simulink model "robots"  (R2018a)
settings: Solver=VariableStepAuto  StartTime=0.0  StopTime=10.0  RelTol=1e-3
undefined symbols (not defined in the file): sigbuilder_block
settings Model: EnablePacing=on  Creator=U500304  LastModifiedBy=U500304

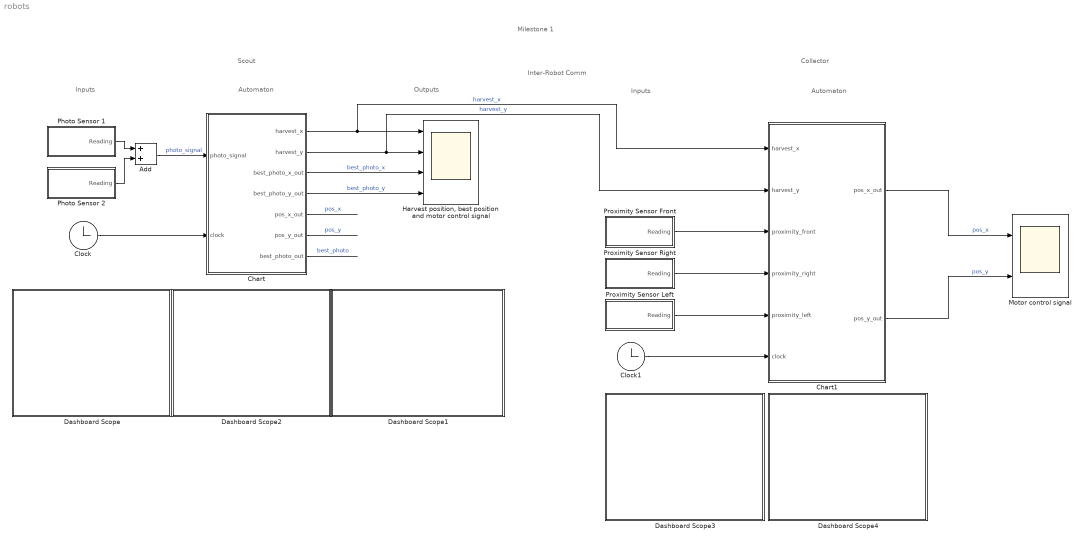
== system robots ==
  note: Inter-Robot
      | Comm
  note: Scout
  note: Milestone 1
  note: Inputs
  note: Automaton
  note: Outputs
  note: Inputs
  note: Collector
  note: Automaton
  Add : Sum
  Chart : Stateflow chart  TreatAsAtomicUnit=on
  Chart1 : Stateflow chart  TreatAsAtomicUnit=on
  Clock : Clock
  Clock1 : Clock
  Dashboard Scope : Subsystem  DialogController=hmiCreateDDGDialog  IsWebBlock=on  mask(MWDashboardBlock){webBlockId=c2b4710b-9c10-441f-91da-978dfb24ecfa, webBlockType=sdiscope, ShowInitialText=on, HMISrcModelName=scout}
      mask prompts: webBlockId "WebBlock Id"; webBlockType "WebBlock Type"; HMISrcModelName "Source Model"
      mask help: SimulinkHMI:dialogs:HMIScopeDialogDesc
      mask Help: helpview([docroot '/mapfiles/simulink.map'], 'hmi_scope')
      mask Display:
      | if strcmp(get_param(bdroot(gcb),'BlockDiagramType'), 'library')
      |     image([(matlabroot) '/toolbox/simulink/hmi/icons/DashboardScope.png']);
      | end
  Dashboard Scope1 : Subsystem  DialogController=hmiCreateDDGDialog  IsWebBlock=on  mask(MWDashboardBlock){webBlockId=2d41d672-6b82-41b2-afbb-9518b0dd4a4f, webBlockType=sdiscope, ShowInitialText=on, HMISrcModelName=scout}
      mask prompts: webBlockId "WebBlock Id"; webBlockType "WebBlock Type"; HMISrcModelName "Source Model"
      mask help: SimulinkHMI:dialogs:HMIScopeDialogDesc
      mask Help: helpview([docroot '/mapfiles/simulink.map'], 'hmi_scope')
      mask Display:
      | if strcmp(get_param(bdroot(gcb),'BlockDiagramType'), 'library')
      |     image([(matlabroot) '/toolbox/simulink/hmi/icons/DashboardScope.png']);
      | end
  Dashboard Scope2 : Subsystem  DialogController=hmiCreateDDGDialog  IsWebBlock=on  mask(MWDashboardBlock){webBlockId=ed7f14d0-e4f2-40fb-83fb-68689640cdf1, webBlockType=sdiscope, ShowInitialText=on, HMISrcModelName=scout}
      mask prompts: webBlockId "WebBlock Id"; webBlockType "WebBlock Type"; HMISrcModelName "Source Model"
      mask help: SimulinkHMI:dialogs:HMIScopeDialogDesc
      mask Help: helpview([docroot '/mapfiles/simulink.map'], 'hmi_scope')
      mask Display:
      | if strcmp(get_param(bdroot(gcb),'BlockDiagramType'), 'library')
      |     image([(matlabroot) '/toolbox/simulink/hmi/icons/DashboardScope.png']);
      | end
  Dashboard Scope3 : Subsystem  DialogController=hmiCreateDDGDialog  IsWebBlock=on  mask(MWDashboardBlock){webBlockId=b30215f1-102d-4ac5-97b6-32221d9819d8, webBlockType=sdiscope, ShowInitialText=on, HMISrcModelName=scout}
      mask prompts: webBlockId "WebBlock Id"; webBlockType "WebBlock Type"; HMISrcModelName "Source Model"
      mask help: SimulinkHMI:dialogs:HMIScopeDialogDesc
      mask Help: helpview([docroot '/mapfiles/simulink.map'], 'hmi_scope')
      mask Display:
      | if strcmp(get_param(bdroot(gcb),'BlockDiagramType'), 'library')
      |     image([(matlabroot) '/toolbox/simulink/hmi/icons/DashboardScope.png']);
      | end
  Dashboard Scope4 : Subsystem  DialogController=hmiCreateDDGDialog  IsWebBlock=on  mask(MWDashboardBlock){webBlockId=4fc18f5f-2100-4ee3-a4cf-c6ec907fe0c9, webBlockType=sdiscope, ShowInitialText=on, HMISrcModelName=scout}
      mask prompts: webBlockId "WebBlock Id"; webBlockType "WebBlock Type"; HMISrcModelName "Source Model"
      mask help: SimulinkHMI:dialogs:HMIScopeDialogDesc
      mask Help: helpview([docroot '/mapfiles/simulink.map'], 'hmi_scope')
      mask Display:
      | if strcmp(get_param(bdroot(gcb),'BlockDiagramType'), 'library')
      |     image([(matlabroot) '/toolbox/simulink/hmi/icons/DashboardScope.png']);
      | end
  "Harvest position, best position and motor control signal" : Scope  NumInputPorts=4
  Motor control signal : Scope  NumInputPorts=2
  Photo Sensor 1 : Subsystem  Tag=STV Subsys  LoadFcn=sigbuilder_block('load');  StartFcn=sigbuilder_block('start');  StopFcn=sigbuilder_block('stop');  ClipboardFcn=sigbuilder_block('clipboard');  mask(Sigbuilder block){tuvar=[0:10]}
      mask help: Simulink:masks:SigbuilderBlock_MD
      mask init:
      | if ~strcmp(get_param(bdroot(gcbh),'SimulationStatus'),'stopped') tuvar = sigbuilder_block('maskInit'); end
      settings: CopyFcn=sigbuilder_block('copy');  DeleteFcn=sigbuilder_block('delete');  ModelCloseFcn=sigbuilder_block('modelClose');  PreSaveFcn=sigbuilder_block('preSave');  PauseFcn=sigbuilder_block('pause');  ContinueFcn=sigbuilder_block('continue');  NameChangeFcn=sigbuilder_block('namechange');  OpenFcn=sigbuilder_block('open',[5.4 30 1141.2 522.6 ]);  CloseFcn=sigbuilder_block('close');
      mask Display: plot(0, 0, 100, 100,[2, 2, 32, 32, 2], [68, 8, 8, 68, 68],[32, 2], [38, 38], [32, 19, 2],[53, 60, 44], [32, 17, 17, 2],[16, 16, 31, 31]);txt = getActiveGroup(gcbh);text(2, 100, txt,'verticalAlignment', 'top');
  Photo Sensor 2 : Subsystem  Tag=STV Subsys  LoadFcn=sigbuilder_block('load');  StartFcn=sigbuilder_block('start');  StopFcn=sigbuilder_block('stop');  ClipboardFcn=sigbuilder_block('clipboard');  mask(Sigbuilder block){tuvar=[0:10]}
      mask help: Simulink:masks:SigbuilderBlock_MD
      mask init:
      | if ~strcmp(get_param(bdroot(gcbh),'SimulationStatus'),'stopped') tuvar = sigbuilder_block('maskInit'); end
      settings: CopyFcn=sigbuilder_block('copy');  DeleteFcn=sigbuilder_block('delete');  ModelCloseFcn=sigbuilder_block('modelClose');  PreSaveFcn=sigbuilder_block('preSave');  PauseFcn=sigbuilder_block('pause');  ContinueFcn=sigbuilder_block('continue');  NameChangeFcn=sigbuilder_block('namechange');  OpenFcn=sigbuilder_block('open',[5.4 30 1141.2 522.6 ]);  CloseFcn=sigbuilder_block('close');
      mask Display: plot(0, 0, 100, 100,[2, 2, 32, 32, 2], [68, 8, 8, 68, 68],[32, 2], [38, 38], [32, 19, 2],[53, 60, 44], [32, 17, 17, 2],[16, 16, 31, 31]);txt = getActiveGroup(gcbh);text(2, 100, txt,'verticalAlignment', 'top');
  Proximity Sensor Front : Subsystem  Tag=STV Subsys  LoadFcn=sigbuilder_block('load');  StartFcn=sigbuilder_block('start');  StopFcn=sigbuilder_block('stop');  ClipboardFcn=sigbuilder_block('clipboard');  mask(Sigbuilder block){tuvar=[0:10]}
      mask help: Simulink:masks:SigbuilderBlock_MD
      mask init:
      | if ~strcmp(get_param(bdroot(gcbh),'SimulationStatus'),'stopped') tuvar = sigbuilder_block('maskInit'); end
      settings: CopyFcn=sigbuilder_block('copy');  DeleteFcn=sigbuilder_block('delete');  ModelCloseFcn=sigbuilder_block('modelClose');  PreSaveFcn=sigbuilder_block('preSave');  PauseFcn=sigbuilder_block('pause');  ContinueFcn=sigbuilder_block('continue');  NameChangeFcn=sigbuilder_block('namechange');  OpenFcn=sigbuilder_block('open',[5.4 30 1141.2 522.6 ]);  CloseFcn=sigbuilder_block('close');
      mask Display: plot(0, 0, 100, 100,[2, 2, 32, 32, 2], [68, 8, 8, 68, 68],[32, 2], [38, 38], [32, 19, 2],[53, 60, 44], [32, 17, 17, 2],[16, 16, 31, 31]);txt = getActiveGroup(gcbh);text(2, 100, txt,'verticalAlignment', 'top');
  Proximity Sensor Left : Subsystem  Tag=STV Subsys  LoadFcn=sigbuilder_block('load');  StartFcn=sigbuilder_block('start');  StopFcn=sigbuilder_block('stop');  ClipboardFcn=sigbuilder_block('clipboard');  mask(Sigbuilder block){tuvar=[0:10]}
      mask help: Simulink:masks:SigbuilderBlock_MD
      mask init:
      | if ~strcmp(get_param(bdroot(gcbh),'SimulationStatus'),'stopped') tuvar = sigbuilder_block('maskInit'); end
      settings: CopyFcn=sigbuilder_block('copy');  DeleteFcn=sigbuilder_block('delete');  ModelCloseFcn=sigbuilder_block('modelClose');  PreSaveFcn=sigbuilder_block('preSave');  PauseFcn=sigbuilder_block('pause');  ContinueFcn=sigbuilder_block('continue');  NameChangeFcn=sigbuilder_block('namechange');  OpenFcn=sigbuilder_block('open',[5.4 30 1141.2 522.6 ]);  CloseFcn=sigbuilder_block('close');
      mask Display: plot(0, 0, 100, 100,[2, 2, 32, 32, 2], [68, 8, 8, 68, 68],[32, 2], [38, 38], [32, 19, 2],[53, 60, 44], [32, 17, 17, 2],[16, 16, 31, 31]);txt = getActiveGroup(gcbh);text(2, 100, txt,'verticalAlignment', 'top');
  Proximity Sensor Right : Subsystem  Tag=STV Subsys  LoadFcn=sigbuilder_block('load');  StartFcn=sigbuilder_block('start');  StopFcn=sigbuilder_block('stop');  ClipboardFcn=sigbuilder_block('clipboard');  mask(Sigbuilder block){tuvar=[0:10]}
      mask help: Simulink:masks:SigbuilderBlock_MD
      mask init:
      | if ~strcmp(get_param(bdroot(gcbh),'SimulationStatus'),'stopped') tuvar = sigbuilder_block('maskInit'); end
      settings: CopyFcn=sigbuilder_block('copy');  DeleteFcn=sigbuilder_block('delete');  ModelCloseFcn=sigbuilder_block('modelClose');  PreSaveFcn=sigbuilder_block('preSave');  PauseFcn=sigbuilder_block('pause');  ContinueFcn=sigbuilder_block('continue');  NameChangeFcn=sigbuilder_block('namechange');  OpenFcn=sigbuilder_block('open',[5.4 30 1141.2 522.6 ]);  CloseFcn=sigbuilder_block('close');
      mask Display: plot(0, 0, 100, 100,[2, 2, 32, 32, 2], [68, 8, 8, 68, 68],[32, 2], [38, 38], [32, 19, 2],[53, 60, 44], [32, 17, 17, 2],[16, 16, 31, 31]);txt = getActiveGroup(gcbh);text(2, 100, txt,'verticalAlignment', 'top');
  wires:
  Chart/6(pos_y_out) -> ?  "pos_y"
  Chart/5(pos_x_out) -> ?  "pos_x"
  Chart/2(harvest_y) -> Chart1/2(harvest_y), "Harvest position, best position and motor control signal"/2  "harvest_y"
  Chart/3(best_photo_x_out) -> "Harvest position, best position and motor control signal"/3  "best_photo_x"
  Chart/1(harvest_x) -> Chart1/1(harvest_x), "Harvest position, best position and motor control signal"/1  "harvest_x"
  Photo Sensor 2/1(Reading) -> Add/2
  Photo Sensor 1/1(Reading) -> Add/1
  Chart/4(best_photo_y_out) -> "Harvest position, best position and motor control signal"/4  "best_photo_y"
  Chart/7(best_photo_out) -> ?  "best_photo"
  Add/1 -> Chart/1(photo_signal)  "photo_signal"
  Clock/1 -> Chart/2(clock)
  Proximity Sensor Front/1(Reading) -> Chart1/3(proximity_front)
  Proximity Sensor Right/1(Reading) -> Chart1/4(proximity_right)
  Proximity Sensor Left/1(Reading) -> Chart1/5(proximity_left)
  Clock1/1 -> Chart1/6(clock)
  Chart1/1(pos_x_out) -> Motor control signal/1  "pos_x"
  Chart1/2(pos_y_out) -> Motor control signal/2  "pos_y"

== system robots/Dashboard Scope ==

== system robots/Dashboard Scope1 ==

== system robots/Dashboard Scope2 ==

== system robots/Dashboard Scope3 ==

== system robots/Dashboard Scope4 ==

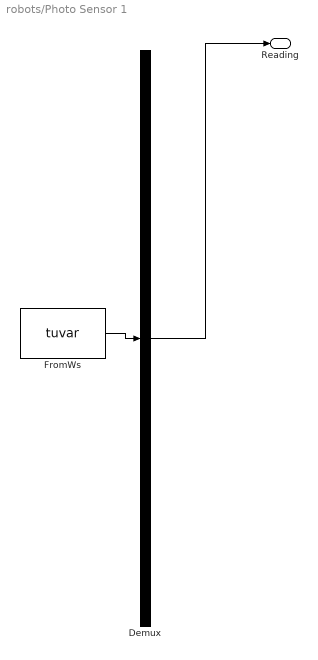
== system robots/Photo Sensor 1 ==
  Demux : Demux  Tag=STV Demux  Outputs=1
  FromWs : FromWorkspace  Tag=STV FromWs  VariableName=tuvar  SampleTime=0
      SigBuilderData=|
      | common.afterFinalStr = 'Extrapolate'
      | common.sampleTime = 0
      | dataSet.timeRange = [0 10]
      | dataSet.name = 'Photo Sensor'
      | sbobj.Groups.Name = 'Photo Sensor'
      | sbobj.Groups.Signals.Name = 'Reading'
      | sbobj.Groups.Signals.XData = [0 6 6 8 8 10]
      | sbobj.Groups.Signals.YData = [0 0 300 300 0 0]
  Reading : Outport  Tag=STV Outport
  wires:
  Demux/1 -> Reading/1
  FromWs/1 -> Demux/1

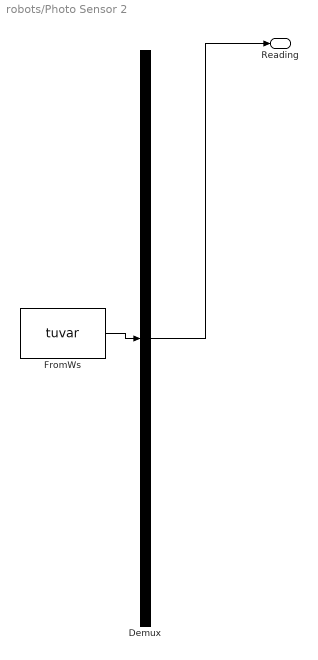
== system robots/Photo Sensor 2 ==
  Demux : Demux  Tag=STV Demux  Outputs=1
  FromWs : FromWorkspace  Tag=STV FromWs  VariableName=tuvar  SampleTime=0
      SigBuilderData=|
      | common.afterFinalStr = 'Extrapolate'
      | common.sampleTime = 0
      | dataSet.timeRange = [0 10]
      | dataSet.name = 'Photo Sensor'
      | sbobj.Groups.Name = 'Photo Sensor'
      | sbobj.Groups.Signals.Name = 'Reading'
      | sbobj.Groups.Signals.XData = [0 2 2 5 5 10]
      | sbobj.Groups.Signals.YData = [0 0 180 180 0 0]
  Reading : Outport  Tag=STV Outport
  wires:
  FromWs/1 -> Demux/1
  Demux/1 -> Reading/1

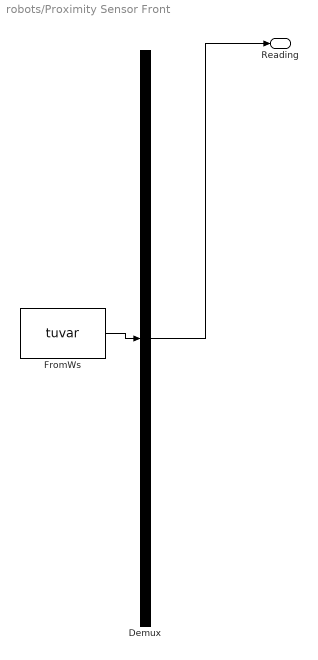
== system robots/Proximity Sensor Front ==
  Demux : Demux  Tag=STV Demux  Outputs=1
  FromWs : FromWorkspace  Tag=STV FromWs  VariableName=tuvar  SampleTime=0
      SigBuilderData=|
      | common.afterFinalStr = 'Extrapolate'
      | common.sampleTime = 0
      | dataSet.timeRange = [0 10]
      | dataSet.name = 'Proximity Front'
      | sbobj.Groups.Name = 'Proximity Front'
      | sbobj.Groups.Signals.Name = 'Reading'
      | sbobj.Groups.Signals.XData = [0 1 8 10]
      | sbobj.Groups.Signals.YData = [10 10 0 0]
  Reading : Outport  Tag=STV Outport
  wires:
  FromWs/1 -> Demux/1
  Demux/1 -> Reading/1

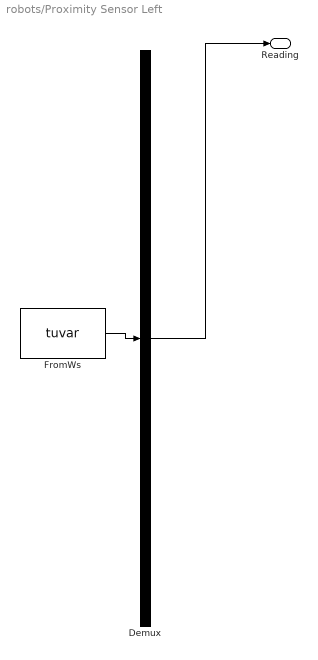
== system robots/Proximity Sensor Left ==
  Demux : Demux  Tag=STV Demux  Outputs=1
  FromWs : FromWorkspace  Tag=STV FromWs  VariableName=tuvar  SampleTime=0
      SigBuilderData=|
      | common.afterFinalStr = 'Extrapolate'
      | common.sampleTime = 0
      | dataSet.timeRange = [0 10]
      | dataSet.name = 'Proximity Left'
      | sbobj.Groups.Name = 'Proximity Left'
      | sbobj.Groups.Signals.Name = 'Reading'
      | sbobj.Groups.Signals.XData = [0 1 2 10]
      | sbobj.Groups.Signals.YData = [2 2 3 8.2]
  Reading : Outport  Tag=STV Outport
  wires:
  FromWs/1 -> Demux/1
  Demux/1 -> Reading/1

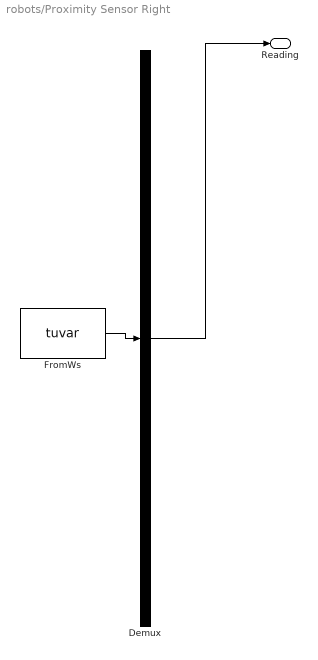
== system robots/Proximity Sensor Right ==
  Demux : Demux  Tag=STV Demux  Outputs=1
  FromWs : FromWorkspace  Tag=STV FromWs  VariableName=tuvar  SampleTime=0
      SigBuilderData=|
      | common.afterFinalStr = 'Extrapolate'
      | common.sampleTime = 0
      | dataSet.timeRange = [0 10]
      | dataSet.name = 'Proximity Right'
      | sbobj.Groups.Name = 'Proximity Right'
      | sbobj.Groups.Signals.Name = 'Reading'
      | sbobj.Groups.Signals.XData = [0 1 10]
      | sbobj.Groups.Signals.YData = [5 4.4 0.55]
  Reading : Outport  Tag=STV Outport
  wires:
  Demux/1 -> Reading/1
  FromWs/1 -> Demux/1

== stateflow chart robots/Chart1 ==
  settings: updateMethod=CONTINUOUS
  state Annoy
    state DriveForward
      du:
      pos_x_dot = 1;
      pos_y_dot = 0;
      pos_x_out = pos_x;
      pos_y_out = pos_y;
    state TurnLeft
      du:
      pos_x_dot = 1;
      pos_y_dot = 0;
      pos_x_out = pos_x;
      pos_y_out = pos_y;
    state TurnRight
      du:
      pos_x_dot = 1;
      pos_y_dot = 0;
      pos_x_out = pos_x;
      pos_y_out = pos_y;
    note: Tries to annoy other robots by pushing them using proximity sensor readings
    (default) -> Annoy.DriveForward
    TurnLeft -> Annoy.DriveForward [order 2] : [proximity_front < proximity_left]
    TurnRight -> Annoy.DriveForward [order 2] : [proximity_front < proximity_right]
    Annoy.DriveForward -> TurnRight [order 2] : [proximity_right < proximity_front]
    Annoy.DriveForward -> TurnLeft [order 1] : [proximity_left < proximity_front]
    TurnLeft -> TurnRight [order 1] : [proximity_right < proximity_left]
    TurnRight -> TurnLeft [order 1] : [proximity_left < proximity_right]
  state Harvest
    state DriveForward
      du:
      pos_x_dot = 0;
      pos_y_dot = 1;
      pos_x_out = pos_x;
      pos_y_out = pos_y;
    note: Drives to the given location of light
    (default) -> Harvest.DriveForward
  (default) -> Annoy : {
      | pos_x = 0;
      | pos_y = 0'
      | }
  Annoy -> Harvest : [harvest_x > -1 && harvest_y > -1]
  data: harvest_x input; harvest_y input; proximity_front input; proximity_right input; proximity_left input; clock input; pos_x local; pos_y local; pos_x_out output; pos_y_out output; target_dir_x local; target_dir_y local
  data pos_x settings: updateMethod=SF_CONTINUOUS_TIME_DATA
  data pos_y settings: updateMethod=SF_CONTINUOUS_TIME_DATA

== stateflow chart robots/Chart ==
  settings: updateMethod=CONTINUOUS
  state Sense [parallel]
    settings: executionOrder=2
    state Dark
    state Light
      en, du:
      harvest_x = pos_x;
      harvest_y = pos_y;
    note: Senses the light and outputs harvest positions
    (default) -> Dark : {
        | best_photo = -1;
        | best_photo_x = -1;
        | best_photo_y = -1;
        | }
    Dark -> Light : [photo_signal > 200]
    Light -> Dark [order 2] : [photo_signal <= 200]
    Light -> Light [order 1] : [photo_signal > best_photo]
        | {best_photo = photo_signal;
        | best_photo_x = pos_x;
        | best_photo_y = pos_y;}
  state Drive [parallel]
    settings: executionOrder=1
    state DriveForward
      du:
      pos_x_dot = 1;
      pos_y_dot = 2;
      pos_x_out = pos_x;
      pos_y_out = pos_y;
    note: Calculates robot's position based on wheel movements
    (default) -> DriveForward : {
        | pos_x = 0;
        | pos_y = 0'
        | }
  state Clock [parallel]
    settings: executionOrder=3
    state Report
      en:
      best_photo_out = best_photo;
      best_photo_x_out = best_photo_x;
      best_photo_y_out = best_photo_y;
    state Seeking
      en:
      cycle_start = clock;
    note: Updates the best harvest position and light reading every 2 seconds
    (default) -> Seeking
    Seeking -> Report : [clock - cycle_start >= 2]
    Report -> Seeking
  data: photo_signal input; harvest_x output =-1; harvest_y output =-1; best_photo_x_out output =-1; best_photo_y_out output =-1; pos_x_out output; pos_y_out output; pos_x local; pos_y local; clock input; best_photo_out output =-1; best_photo local =0; best_photo_x local; best_photo_y local; cycle_start local
  data pos_x settings: updateMethod=SF_CONTINUOUS_TIME_DATA
  data pos_y settings: updateMethod=SF_CONTINUOUS_TIME_DATA
